simulink model "model1"  (R2020a)
settings: Solver=VariableStepAuto  StartTime=0.0  StopTime=100  RelTol=1e-3
settings Model: Creator=11196  LastModifiedBy=11196

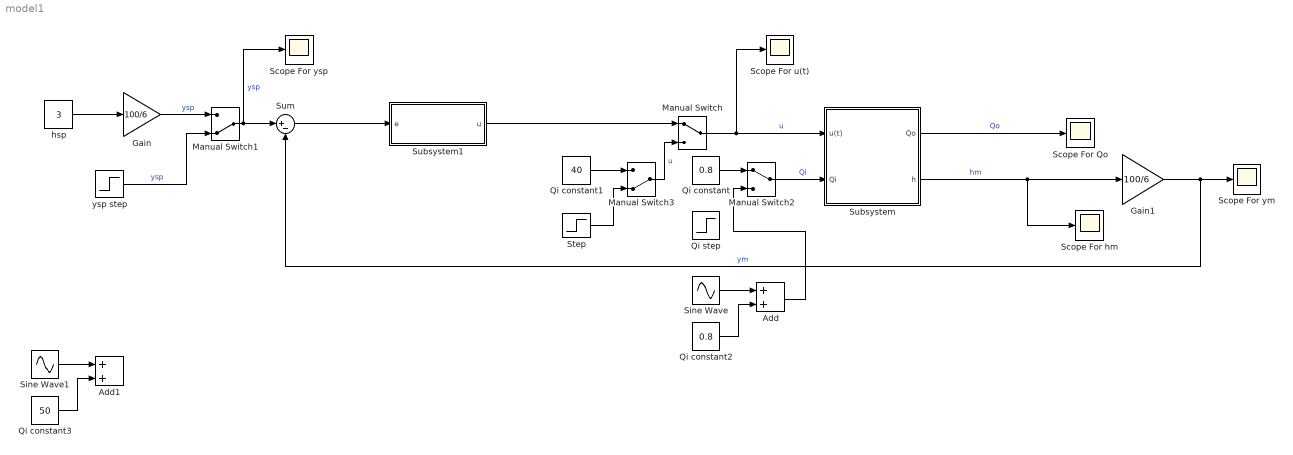
== system model1 ==
  Add : Sum
  Add1 : Sum
  Gain : Gain  Gain=100/6
  Gain1 : Gain  Gain=100/6
  Manual Switch : ManualSwitch
  Manual Switch1 : ManualSwitch  CurrentSetting=0
  Manual Switch2 : ManualSwitch
  Manual Switch3 : ManualSwitch  CurrentSetting=0
  Qi constant : Constant  Value=0.8
  Qi constant1 : Constant  Value=40
  Qi constant2 : Constant  Value=0.8
  Qi constant3 : Constant  Value=50
  Qi step : Step  Time=20  Before=0.8  After=0.96  SampleTime=0
  Scope For Qo : Scope
  Scope For hm : Scope
  Scope For u(t) : Scope
  Scope For ym : Scope
  Scope For ysp : Scope
  Sine Wave : Sin  Amplitude=0.16  Frequency=0.5  SampleTime=0
  Sine Wave1 : Sin  Amplitude=8  Frequency=0.5  SampleTime=0
  Step : Step  Time=20  Before=40  After=48  SampleTime=0
  Subsystem : Subsystem
  Subsystem1 : Subsystem
  Sum : Sum  Inputs=|+-
  hsp : Constant  Value=3
  ysp step : Step  Time=20  Before=50  After=59  SampleTime=0
  wires:
  Subsystem/2(h) -> Scope For hm/1, Gain1/1  "hm"
  Manual Switch/1 -> Scope For u(t)/1, Subsystem/1(u(t))  "u"
  Subsystem/1(Qo) -> Scope For Qo/1  "Qo"
  Manual Switch1/1 -> Scope For ysp/1, Sum/1  "ysp"
  Qi constant/1 -> Manual Switch2/1
  Manual Switch2/1 -> Subsystem/2(Qi)  "Qi"
  Gain1/1 -> Sum/2, Scope For ym/1  "ym"
  hsp/1 -> Gain/1
  Gain/1 -> Manual Switch1/1  "ysp"
  Manual Switch3/1 -> Manual Switch/2  "u"
  Qi constant1/1 -> Manual Switch3/1
  Step/1 -> Manual Switch3/2
  Sum/1 -> Subsystem1/1(e)
  Subsystem1/1(u) -> Manual Switch/1
  Sine Wave/1 -> Add/1
  Qi constant2/1 -> Add/2
  Add/1 -> Manual Switch2/2
  Qi constant3/1 -> Add1/2
  Sine Wave1/1 -> Add1/1
  ysp step/1 -> Manual Switch1/2  "ysp"

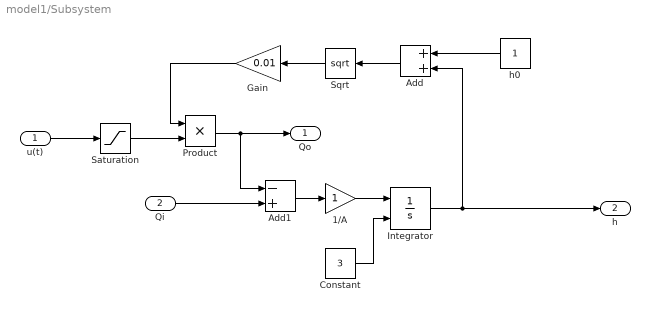
== system model1/Subsystem ==
  u(t) : Inport
  Qi : Inport  Port=2
  1/A : Gain
  Add : Sum
  Add1 : Sum  Inputs=-+
  Constant : Constant  Value=3
  Gain : Gain  Gain=0.01
  Integrator : Integrator  InitialConditionSource=external  InitialCondition=3  LimitOutput=on  UpperSaturationLimit=6  LowerSaturationLimit=0
  Product : Product
  Saturation : Saturate  UpperLimit=100  LowerLimit=0
  Sqrt : Sqrt  SaturateOnIntegerOverflow=on
  h0 : Constant
  Qo : Outport
  h : Outport  Port=2
  wires:
  h0/1 -> Add/1
  Add/1 -> Sqrt/1
  Sqrt/1 -> Gain/1
  Product/1 -> Qo/1, Add1/1
  Qi/1 -> Add1/2
  Add1/1 -> 1/A/1
  1/A/1 -> Integrator/1
  Constant/1 -> Integrator/2
  u(t)/1 -> Saturation/1
  Gain/1 -> Product/1
  Saturation/1 -> Product/2
  Integrator/1 -> h/1, Add/2

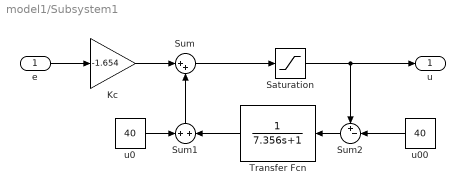
== system model1/Subsystem1 ==
  e : Inport
  Kc : Gain  Gain=-1.654
  Saturation : Saturate  UpperLimit=100  LowerLimit=0
  Sum : Sum  Inputs=|++
  Sum1 : Sum  Inputs=+|+
  Sum2 : Sum  Inputs=+-|
  Transfer Fcn : TransferFcn  Denominator=[7.356 1]
  u0 : Constant  Value=40
  u00 : Constant  Value=40
  u : Outport
  wires:
  e/1 -> Kc/1
  Kc/1 -> Sum/1
  Sum/1 -> Saturation/1
  Saturation/1 -> Sum2/1, u/1
  u00/1 -> Sum2/2
  u0/1 -> Sum1/1
  Sum2/1 -> Transfer Fcn/1
  Transfer Fcn/1 -> Sum1/2
  Sum1/1 -> Sum/2
